simulink model "CF010A_GmTqArbn"  (R2013b)
settings: Solver=FixedStepDiscrete  SolverMode=SingleTasking  StartTime=0.0  StopTime=1  FixedStep=0.002  RelTol=1e-3
values from neighbouring files (symbols this model uses):
  ARCHGLBPRM_2MILLISEC_SEC_F32 = DataDict.Constant    [CF010A_GmTqArbn_DataDict.m]
  ESCTQCMDOVRLLIM_HWNWTMTR_F32 = DataDict.Constant    [CF010A_GmTqArbn_DataDict.m]
  FINALSLEWLWRLIM_HWNWTMTRPERSEC_F32 = DataDict.Constant    [CF010A_GmTqArbn_DataDict.m]
  GmTqArbnApaAssiScaEna = DataDict.Calibration    [CF010A_GmTqArbn_DataDict.m]
  GmTqArbnApaDampgScaEna = DataDict.Calibration    [CF010A_GmTqArbn_DataDict.m]
  GmTqArbnApaEnaRate = DataDict.Calibration    [CF010A_GmTqArbn_DataDict.m]
  GmTqArbnApaRtnScaEna = DataDict.Calibration    [CF010A_GmTqArbn_DataDict.m]
  GmTqArbnEscMaxTq = DataDict.Calibration    [CF010A_GmTqArbn_DataDict.m]
  GmTqArbnLkaOutpOvrlUpprLim = DataDict.Calibration    [CF010A_GmTqArbn_DataDict.m]
  GmTqArbnLkaSlewEna = DataDict.Calibration    [CF010A_GmTqArbn_DataDict.m]
  HWTQCMDOVRLLIM_HWNWTMTR_F32 = DataDict.Constant    [CF010A_GmTqArbn_DataDict.m]
  LKACMDHILIM_HWNWTMTR_F32 = DataDict.Constant    [CF010A_GmTqArbn_DataDict.m]
  LKAOUTPOVRLLIM_MOTNWTMTR_F32 = DataDict.Constant    [CF010A_GmTqArbn_DataDict.m]
  LKATQCMDOVRLLIM_HWNWTMTR_F32 = DataDict.Constant    [CF010A_GmTqArbn_DataDict.m]
  MOTTQCMDOVRLLIM_MOTNWTMTR_F32 = DataDict.Constant    [CF010A_GmTqArbn_DataDict.m]
  OUTPCMDHILIM_ULS_F32 = DataDict.Constant    [CF010A_GmTqArbn_DataDict.m]
  OUTPCMDLOWRLIM_ULS_F32 = DataDict.Constant    [CF010A_GmTqArbn_DataDict.m]
  POSNSERVOSMOOTHMINLWRLIM_ULSPERSEC_F32 = DataDict.Constant    [CF010A_GmTqArbn_DataDict.m]
  VELDPTTQOVRLMTRCOFFS_HWNWTMTRPERSEC_F32 = DataDict.Constant    [CF010A_GmTqArbn_DataDict.m]
  VELDPTTQOVRLMTRCTQPERVEHSPD_HWNWTMTRPERSECPERKPH_F32 = DataDict.Constant    [CF010A_GmTqArbn_DataDict.m]
undefined symbols (not defined in the file or in its folder): GmTqArbnEscSt1, GmTqArbnLkaSt1
libraries: NxtrLim x12, simulink x10, NexteerUtilities x8, FixdToFloat x4, NxtrAbslt x3, Fil x2, FloatToFixd x2, BilnrIntrpnMplX x1, NxtrSign x1
(part 1 of 5)
Description:
  | Torque arbitrator module for overlays for GM applications.
  |      This module uses the signals from external modules, other functions, and enable flags from the GMOSH
  |         to determine the amount of input and output torque overlay to apply to SF-01 and SF-04, respectively, and
  |         the amount of scaling to apply to Assist, Return, and Damping.
settings Model: CovMetricSettings=dcmow  CovHTMLOptions=-sRT=1 -aTS=1 -bRG=1 -bTC=1 -hTR=0 -nFC=0 -scm=1 -bcm=1 -xEv=0  covSaveCumulativeToWorkspaceVar=off  CovSaveSingleToWorkspaceVar=off  CovCumulativeReport=on  Creator=HZ32RQ  LastModifiedBy=nz2988
settings SolverCC: AutoInsertRateTranBlk=on  InsertRTBMode=Always
settings DataIOCC: LimitDataPoints=off  SaveFormat=Structure  ReturnWorkspaceOutputs=on
settings OptimizationCC: BlockReduction=off  InlineParams=on  ZeroExternalMemoryAtStartup=off  ZeroInternalMemoryAtStartup=off  OptimizeModelRefInitCode=on  LifeSpan=1
settings DebuggingCC: SignalInfNanChecking=error  SignalRangeChecking=warning  UnderspecifiedInitializationDetection=Simplified  SolverPrmCheckMsg=error  InheritedTsInSrcMsg=error  DiscreteInheritContinuousMsg=error  SingleTaskRateTransMsg=error  TasksWithSamePriorityMsg=error  SigSpecEnsureSampleTimeMsg=error  CheckMatrixSingularityMsg=error  ParameterUnderflowMsg=error  ParameterPrecisionLossMsg=error  ParameterTunabilityLossMsg=error  FixptConstUnderflowMsg=warning  FixptConstOverflowMsg=warning  VectorMatrixConversionMsg=error  SignalLabelMismatchMsg=error  UnconnectedInputMsg=error  UnconnectedOutputMsg=error  UnconnectedLineMsg=error  SFcnCompatibilityMsg=error  UniqueDataStoreMsg=warning  BusObjectLabelMismatch=error  RootOutportRequireBusObject=error  AssertControl=DisableAll  ModelReferenceIOMsg=error  ModelReferenceVersionMismatchMessage=warning  ModelReferenceIOMismatchMessage=error  ModelReferenceCSMismatchMessage=warning  ModelReferenceDataLoggingMessage=error  StateNameClashWarn=warning  StrictBusMsg=ErrorOnBusTreatedAsVector  NonBusSignalsTreatedAsBus=error  SFUnexpectedBacktrackingDiag=error  SFInvalidInputDataAccessInChartInitDiag=error  SFNoUnconditionalDefaultTransitionDiag=error  SFTransitionOutsideNaturalParentDiag=error  SFUnconditionalTransitionShadowingDiag=error  SFUndirectedBroadcastEventsDiag=error
settings ModelReferenceCC: ModelReferenceNumInstancesAllowed=Single
settings RTWCC: SystemTargetFile=autosar.tlc  GenCodeOnly=on  TemplateMakefile=ert_default_tmf  Description=AUTOSAR  GenerateReport=on  ProcessScript=autosar_make_rtw_hook  LaunchReport=on
settings CodeAppCC: GenerateComments=off  IgnoreCustomStorageClasses=off  CustomSymbolStrType=$N$R$M  CustomSymbolStrBlkIO=$N$M  SimulinkBlockComments=off
settings STFCustomTargetCC: ParMdlRefBuildCompliant=on  CompOptLevelCompliant=on  IncludeMdlTerminateFcn=off  CombineOutputUpdateFcns=on  SuppressErrorStatus=on  ERTFirstTimeCompliant=on  ERTCustomFileBanners=on  SupportNonFinite=off  SupportComplex=off  SupportContinuousTime=off  SupportNonInlinedSFcns=off  MATLABClassNameForMDSCustomization=Simulink.SoftwareTarget.ERTCustomization  AutosarCompliant=on  GRTInterface=off  SystemTargetFile=autosar.tlc
settings ERTTargetCC: CodeReplacementLibrary=ANSI_C  ConcurrentExecutionCompliant=off  IncludeMdlTerminateFcn=off  SuppressErrorStatus=on  SupportNonFinite=off  SupportComplex=off  ModelStepFunctionPrototypeControlCompliant=off  CPPClassGenCompliant=off  AutosarCompliant=on  InlinedParameterPlacement=NonHierarchical  ERTCustomFileTemplate=example_file_process.tlc  EnableUserReplacementTypes=on

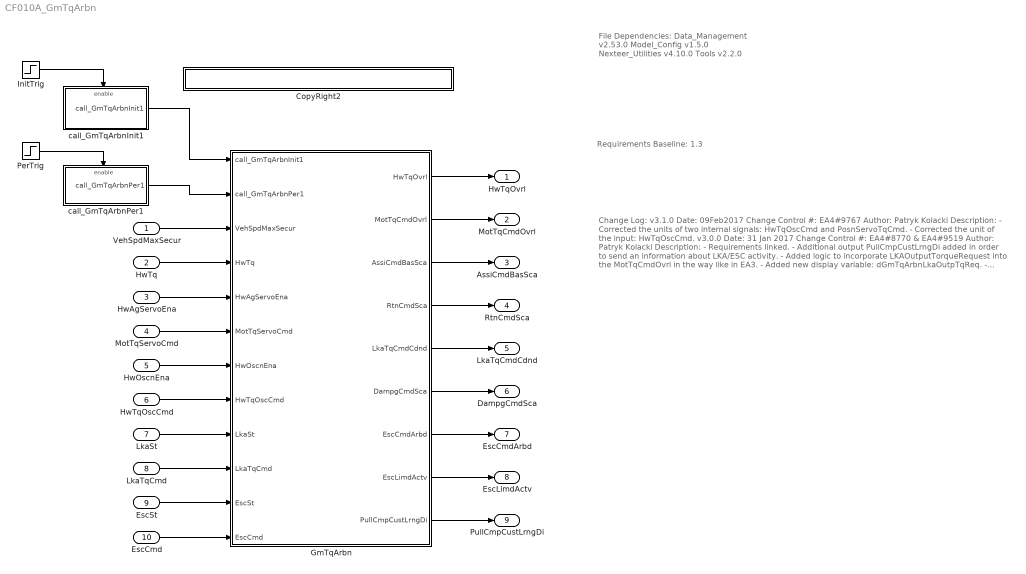
== system CF010A_GmTqArbn ==
  note: File Dependencies:
      |
      | Data_Management v2.53.0
      | Model_Config v1.5.0
      | Nexteer_Utilities v4.10.0
      | Tools v2.2.0
  note: Requirements Baseline: 1.3
  note: Change Log:
      |
      | v3.1.0
      | Date: 09Feb2017
      | Change Control #: EA4#9767
      | Author: Patryk Kolacki
      | Description:
      | - Corrected the units of two internal signals: HwTqOscCmd and PosnServoTqCmd.
      | - Corrected the unit of the input: HwTqOscCmd.
      |
      | v3.0.0
      | Date: 31 Jan 2017
      | Change Control #: EA4#8770 & EA4#9519
      | Author: Patryk Kolacki
      | Description:
      | - Requirements linked.
      | - Additional output PullCmpCustLrngDi added in order to send an information about LKA/ESC activity.
      | - Added logic to incorporate LKAOutputTorqueRequest into the MotTqCmdOvrl in the way like in EA3.
      | - Added new display variable: dGmTqArbnLkaOutpTqReq.
      | - Added following constants: LKAOUTPOVRLLIM_MOTNWTMTR_F32.
      | - Deleted following constants: ESCCMDACTV_CNT_U08 and ESCCMDTMPLIMD_CNT_U08.
      | - Changed the type of LkaSt and EscSt from uint8 to enumerations.
      | - Added following calibrations: GmTqArbnLkaOutpOvrlUpprLim, GmTqArbnLkaOutpOvrlX,
      |   GmTqArbnLkaOutpOvrlY. Precision of the tables has been chaned fro u8p8 to u4p12 comparing to existing
      |   in EA3 solution.
      | - Added following imported calibration: SysGlbPrmVehSpdBilnrSeln.
      | - Changed the ranges of ApaSmotngHwTqLpFil.FilSt and ApaSmotngHwTqLpFil.FilGain
      | - Changed the range of DesLkaTqCmdRateLim (inaccurate in the previous version).
      | - Changed the name of two internal signals: PosnServoTqCmd and OutpTqOvrlCmd.
      | - Corrected logic of obtaining the value of DesLKATqCmd.
      |
      | v2.2.0
      | Date: 19Aug2016
      | Change Control #: EAX#6887
      | Author: Siva
      | Description:
      | - Removed condition "Handwheel Angle Servo Enable = true' for setting Desired LKA Torque Command to Zero
      |   in Determine Desired Value subsystem.
      | - Monotony for 'GmTqArbnLkaSlewY' calibration has been set to 'None' and the Initial value of calibration has
      |   been set to [3  3  3  3  3  3] instead of [12  11  9  7  5  3].
      |
      |
      | V 2.1.0
      | Date: 08June2016
      | Change Control#: EA4#5925/5926
      | Author: Lucas Bowman
      | Description:
      | -Swapped 0 and ESCTqCmd in CAN Conditioning
      | -Changed value of VELDPTTQOVRLMTRCTQPERVEHSPD_HWNWTMTRPERSECPERKPH_F32 to -7/120
      | -Changed background color in all components to white except for GoTo Flags
      | -Eliminated cross wires and unnecessary GoTo flags
      | -Created labels for wires that are associated with temporary varibles in C file
      |
      | V 2.0.0
      | Date: 04April2016
      | Change Control #: EA4#8765
      | Author: Ting Zhan
      | Description:
      | -Replaced Input signal HwTqOscSt with HwOscnEna
      |
      | V 1.1.0
      | Date: 05Jan2016
      | Change Control #: EA4#3623
      | Author: Hemlata Kamble
      | Description:
      | Following issues mentioned in anomaly CR2143 fixed
      | 1. MtrTqServoSmotngEna name changed to HwAgServoEna
      | and corrected Motor Tq servo command signal name.
      | 2. Trig functions updated for Init and Periodic
      | 3.  PIM Variable name corrected
      | 4. Data type of the Constants used were set to 'double' which
      | are now changed to datatype 'single'
      | 5. Removed incorrect links to requirements in model
      | 6. DD is modified to fix the verify_DD tool errors.
      |
      | V 1.0.0
      | Date: 12Aug2015
      | Change Control #: EA4#1687
      | Author: Qi Wang
      | Description:
      | - Initial release based on EA3 v003
  VehSpdMaxSecur : Inport
  HwTq : Inport  Port=2
  HwAgServoEna : Inport  Port=3
  MotTqServoCmd : Inport  Port=4
  HwOscnEna : Inport  Port=5
  HwTqOscCmd : Inport  RequirementInfo={} %GIDa_71ea23b4_56ba_4dec_a781_aee4be0548fb  Port=6
  LkaSt : Inport  Port=7
  LkaTqCmd : Inport  Port=8
  EscSt : Inport  Port=9
  EscCmd : Inport  Port=10
  CopyRight2 : Subsystem  Description=|  mask(Copyright Information){none=on}
      | Copyright info block.                                               
      |                                                                     
      | Place copyright information at the top of every subsystem in design.
      mask prompts: none "No parameters"
      mask help: Place copyright information at the top of every subsystem in design.
      mask Display:
      | NxtrConf = 'Nexteer Confidential';
      | 
      | sys = bdroot; %handle for the current model ("system")
      | first = get_param(sys,'Created');
      | first = first(end-3:end);  %year is last four digits
      | 
      | last = get_param(sys,'LastModifiedDate');
      | if isempty(last)
      |     last = datestr(now,'yyyy');
      | else
      |     last = last(end-3:end);
      | end
      | 
      | if strcmp(first,last)
      |     fprintf('%s -- Copyright %s Nexteer',NxtrConf,first)
      | else
      |     fprintf('%s -- %s%s- %s Nexteer',NxtrConf,char(169),first,last)
      | end
  GmTqArbn : Subsystem
  InitTrig : Step  Time=0.01  Before=1  After=0  SampleTime=0.002
  PerTrig : Step  Time=0.01  SampleTime=0.002
  call_GmTqArbnInit1 : Subsystem  TreatAsAtomicUnit=on
  call_GmTqArbnPer1 : Subsystem  RequirementInfo={} %GIDa_436603c1_ed74_4b99_9aa3_2b152f4c86b9  TreatAsAtomicUnit=on
  HwTqOvrl : Outport
  MotTqCmdOvrl : Outport  Port=2
  AssiCmdBasSca : Outport  Port=3
  RtnCmdSca : Outport  Port=4
  LkaTqCmdCdnd : Outport  Port=5
  DampgCmdSca : Outport  Port=6
  EscCmdArbd : Outport  Port=7
  EscLimdActv : Outport  Port=8
  PullCmpCustLrngDi : Outport  RequirementInfo="{}  %GIDa_53d8df37_3745_4faf_b06d_236ddfd9b0cb"  Port=9
  wires:
  VehSpdMaxSecur/1 -> GmTqArbn/3(VehSpdMaxSecur)
  HwTq/1 -> GmTqArbn/4(HwTq)
  HwAgServoEna/1 -> GmTqArbn/5(HwAgServoEna)
  MotTqServoCmd/1 -> GmTqArbn/6(MotTqServoCmd)
  HwOscnEna/1 -> GmTqArbn/7(HwOscnEna)
  HwTqOscCmd/1 -> GmTqArbn/8(HwTqOscCmd)
  LkaSt/1 -> GmTqArbn/9(LkaSt)
  LkaTqCmd/1 -> GmTqArbn/10(LkaTqCmd)
  EscSt/1 -> GmTqArbn/11(EscSt)
  EscCmd/1 -> GmTqArbn/12(EscCmd)
  GmTqArbn/1(HwTqOvrl) -> HwTqOvrl/1
  GmTqArbn/2(MotTqCmdOvrl) -> MotTqCmdOvrl/1
  GmTqArbn/3(AssiCmdBasSca) -> AssiCmdBasSca/1
  GmTqArbn/4(RtnCmdSca) -> RtnCmdSca/1
  GmTqArbn/5(LkaTqCmdCdnd) -> LkaTqCmdCdnd/1
  GmTqArbn/6(DampgCmdSca) -> DampgCmdSca/1
  GmTqArbn/7(EscCmdArbd) -> EscCmdArbd/1
  GmTqArbn/8(EscLimdActv) -> EscLimdActv/1
  call_GmTqArbnInit1/1(call_GmTqArbnInit1) -> GmTqArbn/1(call_GmTqArbnInit1)
  PerTrig/1 -> call_GmTqArbnPer1/Enable
  call_GmTqArbnPer1/1(call_GmTqArbnPer1) -> GmTqArbn/2(call_GmTqArbnPer1)
  InitTrig/1 -> call_GmTqArbnInit1/Enable
  GmTqArbn/9(PullCmpCustLrngDi) -> PullCmpCustLrngDi/1

== system CF010A_GmTqArbn/CopyRight2 ==

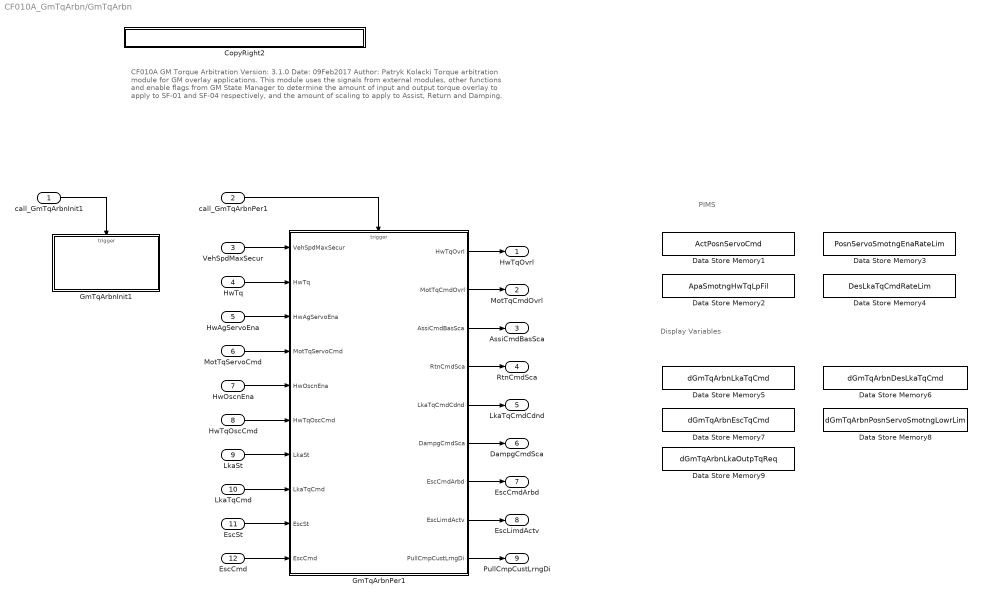
== system CF010A_GmTqArbn/GmTqArbn ==
  note: PIMS
  note: Display Variables
  note: CF010A GM Torque Arbitration
      | Version: 3.1.0      Date: 09Feb2017
      | Author: Patryk Kolacki
      |
      | Torque arbitration module for GM overlay applications.
      | This module uses the signals from external modules, other functions and enable flags from GM State Manager
      | to determine the amount of input and output torque overlay to apply to SF-01 and SF-04 respectively, and the
      | amount of scaling to apply to Assist, Return and Damping.
  call_GmTqArbnInit1 : Inport
  call_GmTqArbnPer1 : Inport  Port=2
  VehSpdMaxSecur : Inport  RequirementInfo="{'linktype_rmi_doors' '0000c6e3 (/E-STEER Core/SubSystem Specifications/Customer Functions - EA4/GM/CF010A GM Torque Arbitrator)' '#CF010A_27' 'true' 'REQ:  CF010A_27' '' } %GIDa_6be114a1_62a0_4d32_aa36_9ad3154e9bd9"  Port=3
  HwTq : Inport  RequirementInfo="{'linktype_rmi_doors' '0000c6e3 (/E-STEER Core/SubSystem Specifications/Customer Functions - EA4/GM/CF010A GM Torque Arbitrator)' '#CF010A_37' 'true' 'REQ:  CF010A_37' '' } %GIDa_2816bad6_3de2_46fa_8d92_2179932feea6"  Port=4
  HwAgServoEna : Inport  RequirementInfo="{'linktype_rmi_doors' '0000c6e3 (/E-STEER Core/SubSystem Specifications/Customer Functions - EA4/GM/CF010A GM Torque Arbitrator)' '#CF010A_38' 'true' 'REQ:  CF010A_38' '' } %GIDa_3e1f97a3_3ca3_4501_b24a_a7c2cef64b8f"  Port=5
  MotTqServoCmd : Inport  RequirementInfo="{'linktype_rmi_doors' '0000c6e3 (/E-STEER Core/SubSystem Specifications/Customer Functions - EA4/GM/CF010A GM Torque Arbitrator)' '#CF010A_41' 'true' 'REQ:  CF010A_41' '' } %GIDa_266a0f77_abbd_494e_bd95_30b6080ab0ba"  Port=6
  HwOscnEna : Inport  RequirementInfo="{'linktype_rmi_doors' '0000c6e3 (/E-STEER Core/SubSystem Specifications/Customer Functions - EA4/GM/CF010A GM Torque Arbitrator)' '#CF010A_43' 'true' 'REQ:  CF010A_43' '' } %GIDa_ae8295f5_6e09_4554_bae7_a39f3185db44"  Port=7
  HwTqOscCmd : Inport  RequirementInfo="{'linktype_rmi_doors' '0000c6e3 (/E-STEER Core/SubSystem Specifications/Customer Functions - EA4/GM/CF010A GM Torque Arbitrator)' '#CF010A_42' 'true' 'REQ:  CF010A_42' '' } %GIDa_603f7c7c_5471_4161_9d84_9eeff5db9061"  Port=8
  LkaSt : Inport  RequirementInfo="{'linktype_rmi_doors' '0000c6e3 (/E-STEER Core/SubSystem Specifications/Customer Functions - EA4/GM/CF010A GM Torque Arbitrator)' '#CF010A_39' 'true' 'REQ:  CF010A_39' '' } %GIDa_308ade94_ba38_409e_a917_d36a285797f0"  Port=9
  LkaTqCmd : Inport  RequirementInfo="{'linktype_rmi_doors' '0000c6e3 (/E-STEER Core/SubSystem Specifications/Customer Functions - EA4/GM/CF010A GM Torque Arbitrator)' '#CF010A_40' 'true' 'REQ:  CF010A_40' '' } %GIDa_bd7b87e9_c6f6_4ed5_82c5_5bdf41894295"  Port=10
  EscSt : Inport  RequirementInfo="{'linktype_rmi_doors' '0000c6e3 (/E-STEER Core/SubSystem Specifications/Customer Functions - EA4/GM/CF010A GM Torque Arbitrator)' '#CF010A_44' 'true' 'REQ:  CF010A_44' '' } %GIDa_b23dc8aa_7d1f_4ac1_aa04_62dd0206bd6a"  Port=11
  EscCmd : Inport  RequirementInfo="{'linktype_rmi_doors' '0000c6e3 (/E-STEER Core/SubSystem Specifications/Customer Functions - EA4/GM/CF010A GM Torque Arbitrator)' '#CF010A_45' 'true' 'REQ:  CF010A_45' '' } %GIDa_3616b8f1_9890_468f_b046_f6f89285dccb"  Port=12
  CopyRight2 : Subsystem  Description=|  mask(Copyright Information){none=on}
      | Copyright info block.                                               
      |                                                                     
      | Place copyright information at the top of every subsystem in design.
      mask prompts: none "No parameters"
      mask help: Place copyright information at the top of every subsystem in design.
      mask Display:
      | NxtrConf = 'Nexteer Confidential';
      | 
      | sys = bdroot; %handle for the current model ("system")
      | first = get_param(sys,'Created');
      | first = first(end-3:end);  %year is last four digits
      | 
      | last = get_param(sys,'LastModifiedDate');
      | if isempty(last)
      |     last = datestr(now,'yyyy');
      | else
      |     last = last(end-3:end);
      | end
      | 
      | if strcmp(first,last)
      |     fprintf('%s -- Copyright %s Nexteer',NxtrConf,first)
      | else
      |     fprintf('%s -- %s%s- %s Nexteer',NxtrConf,char(169),first,last)
      | end
  Data Store Memory1 : DataStoreMemory  DataStoreName=ActPosnServoCmd  StateMustResolveToSignalObject=on
  Data Store Memory2 : DataStoreMemory  DataStoreName=ApaSmotngHwTqLpFil  InitialValue=[]  StateMustResolveToSignalObject=on
  Data Store Memory3 : DataStoreMemory  DataStoreName=PosnServoSmotngEnaRateLim  StateMustResolveToSignalObject=on
  Data Store Memory4 : DataStoreMemory  DataStoreName=DesLkaTqCmdRateLim  StateMustResolveToSignalObject=on
  Data Store Memory5 : DataStoreMemory  DataStoreName=dGmTqArbnLkaTqCmd  StateMustResolveToSignalObject=on
  Data Store Memory6 : DataStoreMemory  DataStoreName=dGmTqArbnDesLkaTqCmd  StateMustResolveToSignalObject=on
  Data Store Memory7 : DataStoreMemory  DataStoreName=dGmTqArbnEscTqCmd  StateMustResolveToSignalObject=on
  Data Store Memory8 : DataStoreMemory  DataStoreName=dGmTqArbnPosnServoSmotngLowrLim  StateMustResolveToSignalObject=on
  Data Store Memory9 : DataStoreMemory  DataStoreName=dGmTqArbnLkaOutpTqReq  StateMustResolveToSignalObject=on
  GmTqArbnInit1 : Subsystem
  GmTqArbnPer1 : Subsystem
  HwTqOvrl : Outport  RequirementInfo="{'linktype_rmi_doors' '0000c6e3 (/E-STEER Core/SubSystem Specifications/Customer Functions - EA4/GM/CF010A GM Torque Arbitrator)' '#CF010A_28' 'true' 'REQ:  CF010A_28' '' } %GIDa_8c5b9742_5c0b_462e_bd72_c17991cb4775"
  MotTqCmdOvrl : Outport  RequirementInfo="{'linktype_rmi_doors' '0000c6e3 (/E-STEER Core/SubSystem Specifications/Customer Functions - EA4/GM/CF010A GM Torque Arbitrator)' '#CF010A_46' 'true' 'REQ:  CF010A_46' '' } %GIDa_00513e15_f241_4486_ae25_adf204a1c6be"  Port=2
  AssiCmdBasSca : Outport  RequirementInfo="{'linktype_rmi_doors' '0000c6e3 (/E-STEER Core/SubSystem Specifications/Customer Functions - EA4/GM/CF010A GM Torque Arbitrator)' '#CF010A_47' 'true' 'REQ:  CF010A_47' '' } %GIDa_9b35394b_4131_4608_84d9_717f18a47ee7"  Port=3
  RtnCmdSca : Outport  RequirementInfo="{'linktype_rmi_doors' '0000c6e3 (/E-STEER Core/SubSystem Specifications/Customer Functions - EA4/GM/CF010A GM Torque Arbitrator)' '#CF010A_48' 'true' 'REQ:  CF010A_48' '' } %GIDa_4a472417_6f5f_4b0d_88e4_ad9a43cb4e05"  Port=4
  LkaTqCmdCdnd : Outport  RequirementInfo="{'linktype_rmi_doors' '0000c6e3 (/E-STEER Core/SubSystem Specifications/Customer Functions - EA4/GM/CF010A GM Torque Arbitrator)' '#CF010A_50' 'true' 'REQ:  CF010A_50' '' } %GIDa_4708c231_0823_4843_953b_1d30a403beb7"  Port=5
  DampgCmdSca : Outport  RequirementInfo="{'linktype_rmi_doors' '0000c6e3 (/E-STEER Core/SubSystem Specifications/Customer Functions - EA4/GM/CF010A GM Torque Arbitrator)' '#CF010A_49' 'true' 'REQ:  CF010A_49' '' } %GIDa_ff68e929_77fd_41ec_ad07_b9c40fc9c43d"  Port=6
  EscCmdArbd : Outport  RequirementInfo="{'linktype_rmi_doors' '0000c6e3 (/E-STEER Core/SubSystem Specifications/Customer Functions - EA4/GM/CF010A GM Torque Arbitrator)' '#CF010A_51' 'true' 'REQ:  CF010A_51' '' } %GIDa_ab7ffc2a_b93c_4013_89bd_4cdb42e1f9c7"  Port=7
  EscLimdActv : Outport  RequirementInfo="{'linktype_rmi_doors' '0000c6e3 (/E-STEER Core/SubSystem Specifications/Customer Functions - EA4/GM/CF010A GM Torque Arbitrator)' '#CF010A_52' 'true' 'REQ:  CF010A_52' '' } %GIDa_513f6eac_2aab_44ee_9a86_6cf40e00f338"  Port=8
  PullCmpCustLrngDi : Outport  RequirementInfo="{'linktype_rmi_doors' '0000c6e3 (/E-STEER Core/SubSystem Specifications/Customer Functions - EA4/GM/CF010A GM Torque Arbitrator)' '#CF010A_107' 'true' 'REQ:  CF010A_107' '' } %GIDa_065d1219_db73_4639_b709_050f9f857351"  Port=9
  wires:
  VehSpdMaxSecur/1 -> GmTqArbnPer1/1(VehSpdMaxSecur)
  HwTq/1 -> GmTqArbnPer1/2(HwTq)
  HwAgServoEna/1 -> GmTqArbnPer1/3(HwAgServoEna)
  MotTqServoCmd/1 -> GmTqArbnPer1/4(MotTqServoCmd)
  HwOscnEna/1 -> GmTqArbnPer1/5(HwOscnEna)
  HwTqOscCmd/1 -> GmTqArbnPer1/6(HwTqOscCmd)
  LkaSt/1 -> GmTqArbnPer1/7(LkaSt)
  LkaTqCmd/1 -> GmTqArbnPer1/8(LkaTqCmd)
  EscSt/1 -> GmTqArbnPer1/9(EscSt)
  EscCmd/1 -> GmTqArbnPer1/10(EscCmd)
  GmTqArbnPer1/1(HwTqOvrl) -> HwTqOvrl/1
  GmTqArbnPer1/2(MotTqCmdOvrl) -> MotTqCmdOvrl/1
  GmTqArbnPer1/3(AssiCmdBasSca) -> AssiCmdBasSca/1
  GmTqArbnPer1/4(RtnCmdSca) -> RtnCmdSca/1
  GmTqArbnPer1/5(LkaTqCmdCdnd) -> LkaTqCmdCdnd/1
  GmTqArbnPer1/6(DampgCmdSca) -> DampgCmdSca/1
  GmTqArbnPer1/7(EscCmdArbd) -> EscCmdArbd/1
  GmTqArbnPer1/8(EscLimdActv) -> EscLimdActv/1
  call_GmTqArbnPer1/1 -> GmTqArbnPer1/Trigger
  call_GmTqArbnInit1/1 -> GmTqArbnInit1/Trigger
  GmTqArbnPer1/9(PullCmpCustLrngDi) -> PullCmpCustLrngDi/1

== system CF010A_GmTqArbn/call_GmTqArbnInit1 ==
  Enable : EnablePort
  FunctionCallGenerator : simulink/Ports & Subsystems/Function-Call Generator  sample_time=.002  numberOfIterations=1
  Subsystem5 : Subsystem  Description=|  mask(Copyright Information){none=on}
      | Copyright info block.                                               
      |                                                                     
      | Place copyright information at the top of every subsystem in design.
      mask prompts: none "No parameters"
      mask help: Place copyright information at the top of every subsystem in design.
      mask Display:
      | NxtrConf = 'Nexteer Confidential';
      | 
      | sys = bdroot; %handle for the current model ("system")
      | first = get_param(sys,'Created');
      | first = first(end-3:end);  %year is last four digits
      | 
      | last = get_param(sys,'LastModifiedDate');
      | if isempty(last)
      |     last = datestr(now,'yyyy');
      | else
      |     last = last(end-3:end);
      | end
      | 
      | if strcmp(first,last)
      |     fprintf('%s -- Copyright %s Nexteer',NxtrConf,first)
      | else
      |     fprintf('%s -- %s%s- %s Nexteer',NxtrConf,char(169),first,last)
      | end
  call_GmTqArbnInit1 : Outport
  wires:
  FunctionCallGenerator/1 -> call_GmTqArbnInit1/1

== system CF010A_GmTqArbn/call_GmTqArbnPer1 ==
  Enable : EnablePort
  FunctionCallGenerator : simulink/Ports & Subsystems/Function-Call Generator  sample_time=.002  numberOfIterations=1
  Subsystem5 : Subsystem  Description=|  mask(Copyright Information){none=on}
      | Copyright info block.                                               
      |                                                                     
      | Place copyright information at the top of every subsystem in design.
      mask prompts: none "No parameters"
      mask help: Place copyright information at the top of every subsystem in design.
      mask Display:
      | NxtrConf = 'Nexteer Confidential';
      | 
      | sys = bdroot; %handle for the current model ("system")
      | first = get_param(sys,'Created');
      | first = first(end-3:end);  %year is last four digits
      | 
      | last = get_param(sys,'LastModifiedDate');
      | if isempty(last)
      |     last = datestr(now,'yyyy');
      | else
      |     last = last(end-3:end);
      | end
      | 
      | if strcmp(first,last)
      |     fprintf('%s -- Copyright %s Nexteer',NxtrConf,first)
      | else
      |     fprintf('%s -- %s%s- %s Nexteer',NxtrConf,char(169),first,last)
      | end
  call_GmTqArbnPer1 : Outport
  wires:
  FunctionCallGenerator/1 -> call_GmTqArbnPer1/1

== system CF010A_GmTqArbn/GmTqArbn/CopyRight2 ==

== system CF010A_GmTqArbn/GmTqArbn/GmTqArbnInit1 ==
  function : TriggerPort  TriggerType=function-call
  ApaSmotngHwTqLoPassFil : Fil/FilLpInit  Ic=0  Ts=ARCHGLBPRM_2MILLISEC_SEC_F32  Freq=GmTqArbnApaSmotngHwTqLpFilFrq  StVar=ApaSmotngHwTqLpFil
  CopyRight2 : Subsystem  Description=|  mask(Copyright Information){none=on}
      | Copyright info block.                                               
      |                                                                     
      | Place copyright information at the top of every subsystem in design.
      mask prompts: none "No parameters"
      mask help: Place copyright information at the top of every subsystem in design.
      mask Display:
      | NxtrConf = 'Nexteer Confidential';
      | 
      | sys = bdroot; %handle for the current model ("system")
      | first = get_param(sys,'Created');
      | if(isempty(first))
      |     first = datestr(now,'yyyy');
      | else
      |     first = first(end-3:end);  %year is last four digits
      | end
      | 
      | last = get_param(sys,'LastModifiedDate');
      | if isempty(last)
      |     last = datestr(now,'yyyy');
      | else
      |     last = last(end-3:end);
      | end
      | 
      | if strcmp(first,last)
      |     fprintf('%s -- Copyright %s Nexteer',NxtrConf,first)
      | else
      |     fprintf('%s -- %s%s- %s Nexteer',NxtrConf,char(169),first,last)
      | end
